simulink model "MKF_example_sim"  (R2021b)
settings: Solver=FixedStepAuto  StartTime=0.0  StopTime=nT*Ts  FixedStep=Ts  RelTol=1e-3
values from neighbouring files (symbols this model uses):
  A = Model.A    [GPB1_estimation.m]    (also in GPB1_estimation_BT.m; GPB2_estimation.m)
  B = Model.B    [GPB1_estimation_BT.m]
  Bu = Model.Bu    [GPB1_estimation.m]    (also in GPB2_estimation.m; MKFObserverSF_RODD.m = model.B(:, io.u_known); MKFObserverSF_RODD95.m = model.B(:, io.u_known); MKFObserverSPF.m = model.B(:, u_meas))
  C = Model.C    [GPB1_estimation.m]    (also in GPB1_estimation_BT.m; GPB2_estimation.m; MKFObserverA.m = obj.filters{f}.C)
  Du = zeros(ny,nu)    [MKFObserverSF_RODD.m]    (also in MKFObserverSF_RODD95.m; MKFObserverSP_RODD.m)
  n = size(models{1}.A, 1)    [GPB1_update.m]    (also in GPB2_update.m)
  ny = size(models{1}.C, 1)    [GPB1_update.m]    (also in GPB2_update.m; MEKF_observer_RODD.m = size(y_meas,1))
  R = Model.R    [GPB1_estimation.m]    (also in GPB1_estimation_BT.m; GPB2_estimation.m; MEKF_observer_RODD.m = repmat({R}, 1, nj))
  x0 = zeros(n, 1)    [AbstractLinearFilter.m]    (also in KalmanFilter.m; KalmanFilterSS_sfunc.m = obs.xkp1_est; MEKF_observer_RODD.m; MKFObserver.m)
undefined symbols (not defined in the file or in its folder): Discrete, KFF, KFF2, KFFSS, KFFSS2, KFP, KFPSS, MKF1, MKF2, SKF, Time, Ts
libraries: ctrlSharedLib x1
settings Model: Creator=Andre  LastModifiedBy=billtubbs
settings SolverCC: AlgebraicLoopSolver=TrustRegion
settings DataIOCC: ReturnWorkspaceOutputs=off
settings DebuggingCC: SFMachineParentedDataDiag=warning  ArithmeticOperatorsInVariantConditions=warning
settings SFSimCC: SimUseLocalCustomCode=off  CustomCodeUndefinedFunction=UseInterfaceOnly
settings RTWCC: RTWUseLocalCustomCode=off

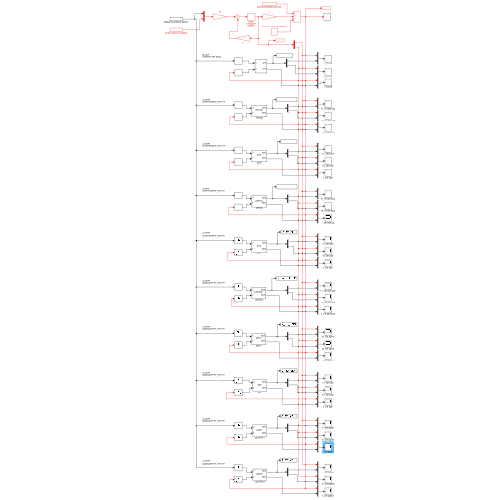
[thumbnail: Simulink's stored preview of the top-level diagram]
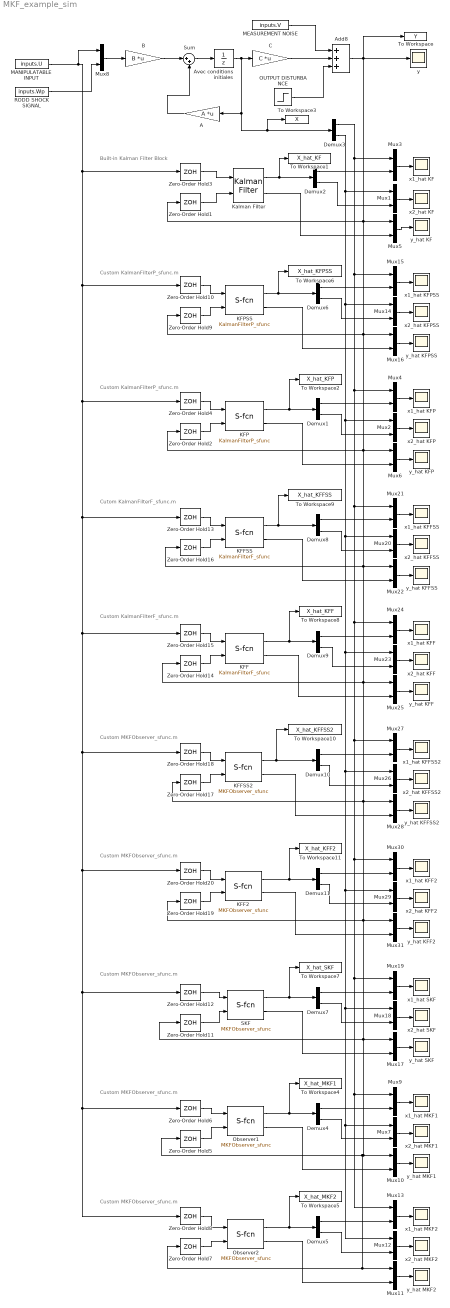
== system MKF_example_sim ==
  note: Built-in
      | Kalman Filter Block
  note: Custom
      | KalmanFilterP_sfunc.m
  note: Custom
      | KalmanFilterP_sfunc.m
  note: Custom
      | MKFObserver_sfunc.m
  note: Cutom
      | KalmanFilterF_sfunc.m
  note: Custom
      | KalmanFilterF_sfunc.m
  note: Custom
      | MKFObserver_sfunc.m
  note: Custom
      | MKFObserver_sfunc.m
  note: Custom
      | MKFObserver_sfunc.m
  note: Custom
      | MKFObserver_sfunc.m
  A : Gain  Gain=A  Multiplication=Matrix(K*u)
  Add8 : Sum  Inputs=+++
  Avec conditions initiales : UnitDelay  InitialCondition=x0  SampleTime=Ts  HasFrameUpgradeWarning=on
  B : Gain  Gain=B  Multiplication=Matrix(K*u)
  C : Gain  Gain=C  Multiplication=Matrix(K*u)
  Demux{1..11} (11 alike) : Demux  Outputs=2
  KFF : M-S-Function  FunctionName=KalmanFilterF_sfunc  Parameters=obs  mask{obs=KFF}
      mask prompts: obs "Observer"
      mask help:
      | Kalman Filter
      |
      | Inputs:
      |  - u : measured process inputs
      |  - y : measured process outputs
      |
      | Outputs:
      |  - xhat : estimate of process states in next time step
      |  - yhat : estimate of process outputs in next time step
      mask Help:
      | <h1>Kalman Filter</h1>
      | 
      | Inputs:
      | <ol>
      | <li>u : measured process inputs (<code>uk</code> argument of update_KF function)
      | <li>y : measured process outputs (<code>yk</code> argument of update_KF function)
      | </ol>
      | 
      | Outputs:
      | <ol>
      | <li>xhat : estimate of process states in next time step (<code>xkp1_est</code> attribute of obs struct)
      | <li>yhat : estimate of process outputs in next time step (<code>ykp1_est</code> of obs struct)
      | </ol>
      | 
      | Use this block to simulate process observers generated by the following MATLAB functions:
      | <ul>
      | <li><code>kalman_filter</code>
      | <li><code>kalman_filter_ss</code>
      | <li><code>luenberger_observer</code>
      | </ul>
      | 
      | <h2>Instructions</h2>
      | 
      | First, generate the observer struct in the MATLAB workspace then pass it to this block in the input field in the block mask. The simulink block will then simulate the observer.  Note that the original MATLAB observer struct will not be updated with the states from the simulation.
      | 
      | The s-functions which can be used with this block:
      | <ul>
      | <li><code>kalman_filter_sfunc</code>
      | <li><code>kalman_filter_ss_sfunc</code>
      | </ul>
      | 
      | To change the s-function, select Mask > Look Under Mask and edit the function name.
      | 
      | <h2>Code repository</h2>
      | <ul>
      | <li><a href="https://github.com/billtubbs/process-observers">https://github.com/billtubbs/process-observers</a>
      | </ul>
      mask Display:
      | port_label('input', 1, 'u')
      | port_label('input', 2, 'y')
      | port_label('output', 1, 'xhat')
      | port_label('output', 2, 'yhat')
      | disp(obs.label)
  KFF2 : M-S-Function  FunctionName=MKFObserver_sfunc  Parameters=obs  mask{obs=KFF2}
      mask prompts: obs "Observer"
      mask help:
      | Multi-Model Process Observer
      |
      | Inputs:
      |  - u : measured process inputs
      |  - y : measured process outputs
      |
      | Outputs:
      |  - xhat : estimate of process states in next time step
      |  - yhat : estimate of process outputs in next time step
      mask Help:
      | <h1>Multi-Model Process Observer</h1>
      | 
      | Inputs:
      | <ol>
      | <li>u : measured process inputs (<code>uk</code> argument of update_KF function)
      | <li>y : measured process outputs (<code>yk</code> argument of update_KF function)
      | </ol>
      | 
      | Outputs:
      | <ol>
      | <li>xhat : estimate of process states in next time step (<code>xkp1_est</code> attribute of obs struct)
      | <li>yhat : estimate of process outputs in next time step (<code>ykp1_est</code> of obs struct)
      | </ol>
      | 
      | Use this block to simulate process observers generated by the following MATLAB functions:
      | <ul>
      | <li><code>kalman_filter</code>
      | <li><code>kalman_filter_ss</code>
      | <li><code>luenberger_observer</code>
      | <li><code>mkf_observer</code>
      | <li><code>mkf_observer_RODD</code>
      | <li><code>mkf_observer_AFMM</code>
      | </ul>
      | 
      | <h2>Instructions</h2>
      | 
      | First, generate the observer struct in the MATLAB workspace then pass it to this block in the input field in the block mask. The simulink block will then simulate the observer.  Note that the original MATLAB observer struct will not be updated with the states from the simulation.
      | 
      | The s-function associated with this block is
      | <ul>
      | <li><code>mkf_observer_sfunc</code>
      | </ul>
      | 
      | <h2>Code repository</h2>
      | <ul>
      | <li><a href="https://github.com/billtubbs/process-observers">https://github.com/billtubbs/process-observers</a>
      | </ul>
      mask Display:
      | port_label('input', 1, 'u')
      | port_label('input', 2, 'y')
      | port_label('output', 1, 'xhat')
      | port_label('output', 2, 'yhat')
      | disp(obs.label)
  KFFSS : M-S-Function  FunctionName=KalmanFilterF_sfunc  Parameters=obs  mask{obs=KFFSS}
      mask prompts: obs "Observer"
      mask help:
      | Kalman Filter
      |
      | Inputs:
      |  - u : measured process inputs
      |  - y : measured process outputs
      |
      | Outputs:
      |  - xhat : estimate of process states in next time step
      |  - yhat : estimate of process outputs in next time step
      mask Help:
      | <h1>Kalman Filter</h1>
      | 
      | Inputs:
      | <ol>
      | <li>u : measured process inputs (<code>uk</code> argument of update_KF function)
      | <li>y : measured process outputs (<code>yk</code> argument of update_KF function)
      | </ol>
      | 
      | Outputs:
      | <ol>
      | <li>xhat : estimate of process states in next time step (<code>xkp1_est</code> attribute of obs struct)
      | <li>yhat : estimate of process outputs in next time step (<code>ykp1_est</code> of obs struct)
      | </ol>
      | 
      | Use this block to simulate process observers generated by the following MATLAB functions:
      | <ul>
      | <li><code>kalman_filter</code>
      | <li><code>kalman_filter_ss</code>
      | <li><code>luenberger_observer</code>
      | </ul>
      | 
      | <h2>Instructions</h2>
      | 
      | First, generate the observer struct in the MATLAB workspace then pass it to this block in the input field in the block mask. The simulink block will then simulate the observer.  Note that the original MATLAB observer struct will not be updated with the states from the simulation.
      | 
      | The s-functions which can be used with this block:
      | <ul>
      | <li><code>kalman_filter_sfunc</code>
      | <li><code>kalman_filter_ss_sfunc</code>
      | </ul>
      | 
      | To change the s-function, select Mask > Look Under Mask and edit the function name.
      | 
      | <h2>Code repository</h2>
      | <ul>
      | <li><a href="https://github.com/billtubbs/process-observers">https://github.com/billtubbs/process-observers</a>
      | </ul>
      mask Display:
      | port_label('input', 1, 'u')
      | port_label('input', 2, 'y')
      | port_label('output', 1, 'xhat')
      | port_label('output', 2, 'yhat')
      | disp(obs.label)
  KFFSS2 : M-S-Function  FunctionName=MKFObserver_sfunc  Parameters=obs  mask{obs=KFFSS2}
      mask prompts: obs "Observer"
      mask help:
      | Multi-Model Process Observer
      |
      | Inputs:
      |  - u : measured process inputs
      |  - y : measured process outputs
      |
      | Outputs:
      |  - xhat : estimate of process states in next time step
      |  - yhat : estimate of process outputs in next time step
      mask Help:
      | <h1>Multi-Model Process Observer</h1>
      | 
      | Inputs:
      | <ol>
      | <li>u : measured process inputs (<code>uk</code> argument of update_KF function)
      | <li>y : measured process outputs (<code>yk</code> argument of update_KF function)
      | </ol>
      | 
      | Outputs:
      | <ol>
      | <li>xhat : estimate of process states in next time step (<code>xkp1_est</code> attribute of obs struct)
      | <li>yhat : estimate of process outputs in next time step (<code>ykp1_est</code> of obs struct)
      | </ol>
      | 
      | Use this block to simulate process observers generated by the following MATLAB functions:
      | <ul>
      | <li><code>kalman_filter</code>
      | <li><code>kalman_filter_ss</code>
      | <li><code>luenberger_observer</code>
      | <li><code>mkf_observer</code>
      | <li><code>mkf_observer_RODD</code>
      | <li><code>mkf_observer_AFMM</code>
      | </ul>
      | 
      | <h2>Instructions</h2>
      | 
      | First, generate the observer struct in the MATLAB workspace then pass it to this block in the input field in the block mask. The simulink block will then simulate the observer.  Note that the original MATLAB observer struct will not be updated with the states from the simulation.
      | 
      | The s-function associated with this block is
      | <ul>
      | <li><code>mkf_observer_sfunc</code>
      | </ul>
      | 
      | <h2>Code repository</h2>
      | <ul>
      | <li><a href="https://github.com/billtubbs/process-observers">https://github.com/billtubbs/process-observers</a>
      | </ul>
      mask Display:
      | port_label('input', 1, 'u')
      | port_label('input', 2, 'y')
      | port_label('output', 1, 'xhat')
      | port_label('output', 2, 'yhat')
      | disp(obs.label)
  KFP : M-S-Function  FunctionName=KalmanFilterP_sfunc  Parameters=obs  mask{obs=KFP}
      mask prompts: obs "Observer"
      mask help:
      | Kalman Filter
      |
      | Inputs:
      |  - u : measured process inputs
      |  - y : measured process outputs
      |
      | Outputs:
      |  - xhat : estimate of process states in next time step
      |  - yhat : estimate of process outputs in next time step
      mask Help:
      | <h1>Kalman Filter</h1>
      | 
      | Inputs:
      | <ol>
      | <li>u : measured process inputs (<code>uk</code> argument of update_KF function)
      | <li>y : measured process outputs (<code>yk</code> argument of update_KF function)
      | </ol>
      | 
      | Outputs:
      | <ol>
      | <li>xhat : estimate of process states in next time step (<code>xkp1_est</code> attribute of obs struct)
      | <li>yhat : estimate of process outputs in next time step (<code>ykp1_est</code> of obs struct)
      | </ol>
      | 
      | Use this block to simulate process observers generated by the following MATLAB functions:
      | <ul>
      | <li><code>kalman_filter</code>
      | <li><code>kalman_filter_ss</code>
      | <li><code>luenberger_observer</code>
      | </ul>
      | 
      | <h2>Instructions</h2>
      | 
      | First, generate the observer struct in the MATLAB workspace then pass it to this block in the input field in the block mask. The simulink block will then simulate the observer.  Note that the original MATLAB observer struct will not be updated with the states from the simulation.
      | 
      | The s-functions which can be used with this block:
      | <ul>
      | <li><code>kalman_filter_sfunc</code>
      | <li><code>kalman_filter_ss_sfunc</code>
      | </ul>
      | 
      | To change the s-function, select Mask > Look Under Mask and edit the function name.
      | 
      | <h2>Code repository</h2>
      | <ul>
      | <li><a href="https://github.com/billtubbs/process-observers">https://github.com/billtubbs/process-observers</a>
      | </ul>
      mask Display:
      | port_label('input', 1, 'u')
      | port_label('input', 2, 'y')
      | port_label('output', 1, 'xhat')
      | port_label('output', 2, 'yhat')
      | disp(obs.label)
  KFPSS : M-S-Function  FunctionName=KalmanFilterP_sfunc  Parameters=obs  mask{obs=KFPSS}
      mask prompts: obs "Observer"
      mask help:
      | Kalman Filter
      |
      | Inputs:
      |  - u : measured process inputs
      |  - y : measured process outputs
      |
      | Outputs:
      |  - xhat : estimate of process states in next time step
      |  - yhat : estimate of process outputs in next time step
      mask Help:
      | <h1>Kalman Filter</h1>
      | 
      | Inputs:
      | <ol>
      | <li>u : measured process inputs (<code>uk</code> argument of update_KF function)
      | <li>y : measured process outputs (<code>yk</code> argument of update_KF function)
      | </ol>
      | 
      | Outputs:
      | <ol>
      | <li>xhat : estimate of process states in next time step (<code>xkp1_est</code> attribute of obs struct)
      | <li>yhat : estimate of process outputs in next time step (<code>ykp1_est</code> of obs struct)
      | </ol>
      | 
      | Use this block to simulate process observers generated by the following MATLAB functions:
      | <ul>
      | <li><code>kalman_filter</code>
      | <li><code>kalman_filter_ss</code>
      | <li><code>luenberger_observer</code>
      | </ul>
      | 
      | <h2>Instructions</h2>
      | 
      | First, generate the observer struct in the MATLAB workspace then pass it to this block in the input field in the block mask. The simulink block will then simulate the observer.  Note that the original MATLAB observer struct will not be updated with the states from the simulation.
      | 
      | The s-functions which can be used with this block:
      | <ul>
      | <li><code>kalman_filter_sfunc</code>
      | <li><code>kalman_filter_ss_sfunc</code>
      | </ul>
      | 
      | To change the s-function, select Mask > Look Under Mask and edit the function name.
      | 
      | <h2>Code repository</h2>
      | <ul>
      | <li><a href="https://github.com/billtubbs/process-observers">https://github.com/billtubbs/process-observers</a>
      | </ul>
      mask Display:
      | port_label('input', 1, 'u')
      | port_label('input', 2, 'y')
      | port_label('output', 1, 'xhat')
      | port_label('output', 2, 'yhat')
      | disp(obs.label)
  Kalman Filter : ctrlSharedLib/Kalman Filter  TimeDomain=Discrete-Time  UseCurrentEstimator=off  ModelSource=Individual A, B, C, D matrices  ModelSourceVariable=G  A=A  B=Bu  C=C  D=Du  NumberOfStates=1  NumberOfInputs=1  NumberOfOutputs=1  InitialEstimateSource=Dialog  X0=[0; 0]  P0=10  UseK=off  UseGH=off  NumberOfProcessNoiseInputs=1  G=Gkf  TimeInvariantG=on  H=Hkf  TimeInvariantH=on  Q=Q  TimeInvariantQ=on  R=R  TimeInvariantR=on  N=zeros(n,ny)  TimeInvariantN=on  AddInputPort=on  AddEnablePort=off  OutputEstimatedY=on  OutputP=off  Ts=Ts
  MANIPULATABLE INPUT : FromWorkspace  VariableName=inputs.U  SampleTime=Ts
  MEASUREMENT NOISE : FromWorkspace  VariableName=inputs.V  SampleTime=Ts
  Mux{1..31} (31 alike) : Mux  Inputs=2
  OUTPUT DISTURBANCE : Step  Time=100  After=0  SampleTime=0
  Observer1 : M-S-Function  FunctionName=MKFObserver_sfunc  Parameters=obs  mask{obs=MKF1}
      mask prompts: obs "Observer"
      mask help:
      | Multi-Model Process Observer
      |
      | Inputs:
      |  - u : measured process inputs
      |  - y : measured process outputs
      |
      | Outputs:
      |  - xhat : estimate of process states in next time step
      |  - yhat : estimate of process outputs in next time step
      mask Help:
      | <h1>Multi-Model Process Observer</h1>
      | 
      | Inputs:
      | <ol>
      | <li>u : measured process inputs (<code>uk</code> argument of update_KF function)
      | <li>y : measured process outputs (<code>yk</code> argument of update_KF function)
      | </ol>
      | 
      | Outputs:
      | <ol>
      | <li>xhat : estimate of process states in next time step (<code>xkp1_est</code> attribute of obs struct)
      | <li>yhat : estimate of process outputs in next time step (<code>ykp1_est</code> of obs struct)
      | </ol>
      | 
      | Use this block to simulate process observers generated by the following MATLAB functions:
      | <ul>
      | <li><code>kalman_filter</code>
      | <li><code>kalman_filter_ss</code>
      | <li><code>luenberger_observer</code>
      | <li><code>mkf_observer</code>
      | <li><code>mkf_observer_RODD</code>
      | <li><code>mkf_observer_AFMM</code>
      | </ul>
      | 
      | <h2>Instructions</h2>
      | 
      | First, generate the observer struct in the MATLAB workspace then pass it to this block in the input field in the block mask. The simulink block will then simulate the observer.  Note that the original MATLAB observer struct will not be updated with the states from the simulation.
      | 
      | The s-function associated with this block is
      | <ul>
      | <li><code>mkf_observer_sfunc</code>
      | </ul>
      | 
      | <h2>Code repository</h2>
      | <ul>
      | <li><a href="https://github.com/billtubbs/process-observers">https://github.com/billtubbs/process-observers</a>
      | </ul>
      mask Display:
      | port_label('input', 1, 'u')
      | port_label('input', 2, 'y')
      | port_label('output', 1, 'xhat')
      | port_label('output', 2, 'yhat')
      | disp(obs.label)
  Observer2 : M-S-Function  FunctionName=MKFObserver_sfunc  Parameters=obs  mask{obs=MKF2}
      mask prompts: obs "Observer"
      mask help:
      | Process Observer
      |
      | Use this block to simulate process observers generated by the following MATLAB functions:
      |  - kalman_filter
      |  - kalman_filter_ss
      |  - luenberger_observer
      |  - mkf_observer
      |  - mkf_observer_RODD
      |  - mkf_observer_AFMM
      mask Help:
      | Process Observer
      | 
      | Use this block to simulate process observers generated by the following MATLAB functions:
      |  - kalman_filter
      |  - kalman_filter_ss
      |  - luenberger_observer
      |  - mkf_observer
      |  - mkf_observer_RODD
      |  - mkf_observer_AFMM
      | 
      | First, generate the observer struct in the MATLAB workspace then pass it to this block in the input field in the block mask. The simulink block will then simulate the observer.  Note that the original MATLAB observer struct will not be updated with the states from the simulation.
      | 
      | The s-function associated with this block is
      |  - mkf_observer_sfunc
      | 
      | Code repository:
      |  - https://github.com/billtubbs/process-observers
      mask Display:
      | port_label('input', 1, 'u')
      | port_label('input', 2, 'y')
      | port_label('output', 1, 'xhat')
      | port_label('output', 2, 'yhat')
      | disp(obs.label)
  RODD SHOCK SIGNAL : FromWorkspace  VariableName=inputs.Wp  SampleTime=Ts
  SKF : M-S-Function  FunctionName=MKFObserver_sfunc  Parameters=obs  mask{obs=SKF}
      mask prompts: obs "Observer"
      mask help:
      | Multi-Model Process Observer
      |
      | Inputs:
      |  - u : measured process inputs
      |  - y : measured process outputs
      |
      | Outputs:
      |  - xhat : estimate of process states in next time step
      |  - yhat : estimate of process outputs in next time step
      mask Help:
      | <h1>Multi-Model Process Observer</h1>
      | 
      | Inputs:
      | <ol>
      | <li>u : measured process inputs (<code>uk</code> argument of update_KF function)
      | <li>y : measured process outputs (<code>yk</code> argument of update_KF function)
      | </ol>
      | 
      | Outputs:
      | <ol>
      | <li>xhat : estimate of process states in next time step (<code>xkp1_est</code> attribute of obs struct)
      | <li>yhat : estimate of process outputs in next time step (<code>ykp1_est</code> of obs struct)
      | </ol>
      | 
      | Use this block to simulate process observers generated by the following MATLAB functions:
      | <ul>
      | <li><code>kalman_filter</code>
      | <li><code>kalman_filter_ss</code>
      | <li><code>luenberger_observer</code>
      | <li><code>mkf_observer</code>
      | <li><code>mkf_observer_RODD</code>
      | <li><code>mkf_observer_AFMM</code>
      | </ul>
      | 
      | <h2>Instructions</h2>
      | 
      | First, generate the observer struct in the MATLAB workspace then pass it to this block in the input field in the block mask. The simulink block will then simulate the observer.  Note that the original MATLAB observer struct will not be updated with the states from the simulation.
      | 
      | The s-function associated with this block is
      | <ul>
      | <li><code>mkf_observer_sfunc</code>
      | </ul>
      | 
      | <h2>Code repository</h2>
      | <ul>
      | <li><a href="https://github.com/billtubbs/process-observers">https://github.com/billtubbs/process-observers</a>
      | </ul>
      mask Display:
      | port_label('input', 1, 'u')
      | port_label('input', 2, 'y')
      | port_label('output', 1, 'xhat')
      | port_label('output', 2, 'yhat')
      | disp(obs.label)
  Sum : Sum  Inputs=|++
  To Workspace : ToWorkspace  VariableName=Y  SaveFormat=Timeseries  SampleTime=-1
  To Workspace1 : ToWorkspace  VariableName=X_hat_KF  SaveFormat=Timeseries  SampleTime=-1
  To Workspace10 : ToWorkspace  VariableName=X_hat_KFFSS2  SaveFormat=Timeseries  SampleTime=-1
  To Workspace11 : ToWorkspace  VariableName=X_hat_KFF2  SaveFormat=Timeseries  SampleTime=-1
  To Workspace2 : ToWorkspace  VariableName=X_hat_KFP  SaveFormat=Timeseries  SampleTime=-1
  To Workspace3 : ToWorkspace  VariableName=X  SaveFormat=Timeseries  SampleTime=-1
  To Workspace4 : ToWorkspace  VariableName=X_hat_MKF1  SaveFormat=Timeseries  SampleTime=-1
  To Workspace5 : ToWorkspace  VariableName=X_hat_MKF2  SaveFormat=Timeseries  SampleTime=-1
  To Workspace6 : ToWorkspace  VariableName=X_hat_KFPSS  SaveFormat=Timeseries  SampleTime=-1
  To Workspace7 : ToWorkspace  VariableName=X_hat_SKF  SaveFormat=Timeseries  SampleTime=-1
  To Workspace8 : ToWorkspace  VariableName=X_hat_KFF  SaveFormat=Timeseries  SampleTime=-1
  To Workspace9 : ToWorkspace  VariableName=X_hat_KFFSS  SaveFormat=Timeseries  SampleTime=-1
  Zero-Order Hold{1..20} (20 alike) : ZeroOrderHold  SampleTime=Ts
  x1_hat KF : Scope
  x1_hat KFF : Scope
  x1_hat KFF2 : Scope
  x1_hat KFFSS : Scope
  x1_hat KFFSS2 : Scope
  x1_hat KFP : Scope
  x1_hat KFPSS : Scope
  x1_hat MKF1 : Scope
  x1_hat MKF2 : Scope
  x1_hat SKF : Scope
  x2_hat KF : Scope
  x2_hat KFF : Scope
  x2_hat KFF2 : Scope
  x2_hat KFFSS : Scope
  x2_hat KFFSS2 : Scope
  x2_hat KFP : Scope
  x2_hat KFPSS : Scope
  x2_hat MKF1 : Scope
  x2_hat MKF2 : Scope
  x2_hat SKF : Scope
  y : Scope
  y_hat KF : Scope
  y_hat KFF : Scope
  y_hat KFF2 : Scope
  y_hat KFFSS : Scope
  y_hat KFFSS2 : Scope
  y_hat KFP : Scope
  y_hat KFPSS : Scope
  y_hat MKF1 : Scope
  y_hat MKF2 : Scope
  y_hat SKF : Scope
  wires:
  A/1 -> Sum/2
  Mux3/1 -> x1_hat KF/1
  Mux1/1 -> x2_hat KF/1
  Sum/1 -> Avec conditions initiales/1
  B/1 -> Sum/1
  OUTPUT DISTURBANCE/1 -> Add8/3
  C/1 -> Add8/2
  MEASUREMENT NOISE/1 -> Add8/1
  Kalman Filter/2 -> Mux5/2
  Mux5/1 -> y_hat KF/1
  Kalman Filter/1 -> To Workspace1/1, Demux2/1
  Demux2/1 -> Mux3/2
  Demux2/2 -> Mux1/2
  Zero-Order Hold3/1 -> Kalman Filter/1
  Zero-Order Hold1/1 -> Kalman Filter/2
  RODD SHOCK SIGNAL/1 -> Mux8/2
  Mux8/1 -> B/1
  Zero-Order Hold4/1 -> KFP/1
  Zero-Order Hold2/1 -> KFP/2
  Mux6/1 -> y_hat KFP/1
  Mux4/1 -> x1_hat KFP/1
  Mux2/1 -> x2_hat KFP/1
  Demux1/1 -> Mux4/2
  Demux1/2 -> Mux2/2
  Avec conditions initiales/1 -> C/1, Demux3/1, To Workspace3/1, A/1
  Demux4/2 -> Mux7/2
  Mux9/1 -> x1_hat MKF1/1
  Observer1/2 -> Mux10/2
  Observer1/1 -> To Workspace4/1, Demux4/1
  Mux7/1 -> x2_hat MKF1/1
  Demux4/1 -> Mux9/2
  Mux10/1 -> y_hat MKF1/1
  Zero-Order Hold6/1 -> Observer1/1
  Zero-Order Hold5/1 -> Observer1/2
  Mux11/1 -> y_hat MKF2/1
  Observer2/1 -> To Workspace5/1, Demux5/1
  Observer2/2 -> Mux11/2
  Mux13/1 -> x1_hat MKF2/1
  Mux12/1 -> x2_hat MKF2/1
  Demux5/1 -> Mux13/2
  Zero-Order Hold8/1 -> Observer2/1
  Demux5/2 -> Mux12/2
  Zero-Order Hold7/1 -> Observer2/2
  Mux16/1 -> y_hat KFPSS/1
  Demux6/1 -> Mux15/2
  Mux15/1 -> x1_hat KFPSS/1
  Demux6/2 -> Mux14/2
  Zero-Order Hold10/1 -> KFPSS/1
  KFPSS/1 -> To Workspace6/1, Demux6/1
  Mux14/1 -> x2_hat KFPSS/1
  KFPSS/2 -> Mux16/2
  Zero-Order Hold9/1 -> KFPSS/2
  KFP/1 -> To Workspace2/1, Demux1/1
  KFP/2 -> Mux6/2
  Demux7/1 -> Mux19/2
  Demux7/2 -> Mux18/2
  Mux17/1 -> y_hat SKF/1
  Mux18/1 -> x2_hat SKF/1
  Zero-Order Hold11/1 -> SKF/2
  Mux19/1 -> x1_hat SKF/1
  SKF/2 -> Mux17/2
  SKF/1 -> To Workspace7/1, Demux7/1
  Zero-Order Hold12/1 -> SKF/1
  Zero-Order Hold14/1 -> KFF/2
  Demux8/1 -> Mux21/2
  KFFSS/1 -> To Workspace9/1, Demux8/1
  Demux9/2 -> Mux23/2
  Demux8/2 -> Mux20/2
  Zero-Order Hold15/1 -> KFF/1
  Zero-Order Hold13/1 -> KFFSS/1
  Mux22/1 -> y_hat KFFSS/1
  Mux23/1 -> x2_hat KFF/1
  Zero-Order Hold16/1 -> KFFSS/2
  Mux20/1 -> x2_hat KFFSS/1
  Mux21/1 -> x1_hat KFFSS/1
  KFF/2 -> Mux25/2
  KFFSS/2 -> Mux22/2
  Mux24/1 -> x1_hat KFF/1
  Demux9/1 -> Mux24/2
  Mux25/1 -> y_hat KFF/1
  KFF/1 -> Demux9/1, To Workspace8/1
  Zero-Order Hold18/1 -> KFFSS2/1
  Zero-Order Hold17/1 -> KFFSS2/2
  KFFSS2/1 -> Demux10/1, To Workspace10/1
  KFFSS2/2 -> Mux28/2
  Mux26/1 -> x2_hat KFFSS2/1
  Mux27/1 -> x1_hat KFFSS2/1
  Add8/1 -> To Workspace/1, Mux31/1, Zero-Order Hold19/1, Zero-Order Hold7/1, Mux11/1, Zero-Order Hold5/1, Mux10/1, Zero-Order Hold11/1, Mux17/1, Zero-Order Hold17/1, Mux28/1, Zero-Order Hold14/1, Mux25/1, Zero-Order Hold16/1, Mux22/1, Zero-Order Hold2/1, Mux6/1, Zero-Order Hold9/1, Mux16/1, Zero-Order Hold1/1, Mux5/1, y/1
  Mux28/1 -> y_hat KFFSS2/1
  MANIPULATABLE INPUT/1 -> Mux8/1, Zero-Order Hold18/1, Zero-Order Hold20/1, Zero-Order Hold8/1, Zero-Order Hold6/1, Zero-Order Hold12/1, Zero-Order Hold15/1, Zero-Order Hold13/1, Zero-Order Hold4/1, Zero-Order Hold10/1, Zero-Order Hold3/1
  Demux10/1 -> Mux27/2
  Demux10/2 -> Mux26/2
  Demux11/2 -> Mux29/2
  Zero-Order Hold20/1 -> KFF2/1
  Demux3/1 -> Mux24/1, Mux27/1, Mux30/1, Mux9/1, Mux13/1, Mux19/1, Mux21/1, Mux4/1, Mux15/1, Mux3/1
  Demux11/1 -> Mux30/2
  Zero-Order Hold19/1 -> KFF2/2
  KFF2/1 -> Demux11/1, To Workspace11/1
  Mux30/1 -> x1_hat KFF2/1
  Mux29/1 -> x2_hat KFF2/1
  Mux31/1 -> y_hat KFF2/1
  KFF2/2 -> Mux31/2
  Demux3/2 -> Mux20/1, Mux23/1, Mux26/1, Mux29/1, Mux7/1, Mux12/1, Mux18/1, Mux2/1, Mux14/1, Mux1/1
